simulink model "P2"  (R2018a)
settings: Solver=VariableStepAuto  StartTime=0.0  StopTime=300  RelTol=1e-3
values from neighbouring files (symbols this model uses):
  n = 5    [Q2.m]
undefined symbols (not defined in the file or in its folder): m
settings Model: Creator=aminrakhsha  LastModifiedBy=whitefox

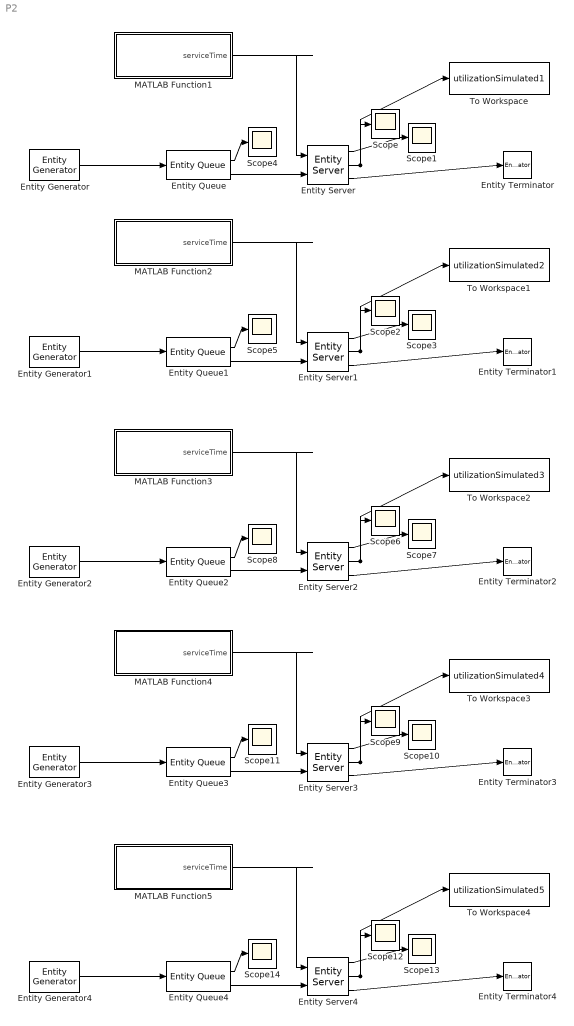
== system P2 ==
  Entity Generator : EntityGenerator  OutputPortMessageModes=m  TimeSource=MATLAB action  Period=5  IntergenerationTimeAction=|  EntityType=Structured  EntityTypeName=Entity
      | persistent counter;
      | if isempty(counter)
      |    counter = 1;
      | end 
      | if counter <= 100
      |     mean=2;
      |     dt = -mean*log(1-rand());
      | else
      |     dt = inf;
      | end
      | counter = counter + 1
  Entity Generator1 : EntityGenerator  OutputPortMessageModes=m  TimeSource=MATLAB action  Period=5  IntergenerationTimeAction=|  EntityType=Structured  EntityTypeName=Entity
      | persistent counter
      | if isempty(counter)
      |    counter = 1;
      | end 
      | if counter <= 100
      |     mean=2;
      |     dt = -mean*log(1-rand());
      | else
      |     dt = inf;
      | end
      | counter = counter + 1
  Entity Generator2 : EntityGenerator  OutputPortMessageModes=m  TimeSource=MATLAB action  Period=5  IntergenerationTimeAction=|  EntityType=Structured  EntityTypeName=Entity
      | persistent counter
      | if isempty(counter)
      |    counter = 1;
      | end 
      | if counter <= 100
      |     mean=2;
      |     dt = -mean*log(1-rand());
      | else
      |     dt = inf;
      | end
      | counter = counter + 1
  Entity Generator3 : EntityGenerator  OutputPortMessageModes=m  TimeSource=MATLAB action  Period=5  IntergenerationTimeAction=|  EntityType=Structured  EntityTypeName=Entity
      | persistent counter
      | if isempty(counter)
      |    counter = 1;
      | end 
      | if counter <= 100
      |     mean=2;
      |     dt = -mean*log(1-rand());
      | else
      |     dt = inf;
      | end
      | counter = counter + 1
  Entity Generator4 : EntityGenerator  OutputPortMessageModes=m  TimeSource=MATLAB action  Period=5  IntergenerationTimeAction=|  EntityType=Structured  EntityTypeName=Entity
      | persistent counter
      | if isempty(counter)
      |    counter = 1;
      | end 
      | if counter <= 100
      |     mean=2;
      |     dt = -mean*log(1-rand());
      | else
      |     dt = inf;
      | end
      | counter = counter + 1
  Entity Queue{,1..4} (5 alike) : EntityQueue  InputPortMessageModes=m  OutputPortMessageModes=n,m  Capacity=inf  AverageWait=on
      settings: OutputPortMap=o2,o5
  Entity Server{,1..4} (5 alike) : EntityServer  InputPortMessageModes=n,m  OutputPortMessageModes=n,n,m  Capacity=1  ServiceTimeSource=Signal port  ServiceTimeAttributeName=Attribute1  ServiceTimeAction=dt = getST(y);  AverageWait=on  Utilization=on
      settings: InputPortMap=u0,u2  OutputPortMap=o4,o5,o9
  Entity Terminator{,1..4} (5 alike) : EntityTerminator  InputPortMessageModes=m
  MATLAB Function1 : MATLAB Function  TreatAsAtomicUnit=on
  MATLAB Function2 : MATLAB Function  TreatAsAtomicUnit=on
  MATLAB Function3 : MATLAB Function  TreatAsAtomicUnit=on
  MATLAB Function4 : MATLAB Function  TreatAsAtomicUnit=on
  MATLAB Function5 : MATLAB Function  TreatAsAtomicUnit=on
  Scope{,1..14} (15 alike) : Scope
  To Workspace : ToWorkspace  VariableName=utilizationSimulated1  SaveFormat=Timeseries  SampleTime=-1
  To Workspace1 : ToWorkspace  VariableName=utilizationSimulated2  SaveFormat=Timeseries  SampleTime=-1
  To Workspace2 : ToWorkspace  VariableName=utilizationSimulated3  SaveFormat=Timeseries  SampleTime=-1
  To Workspace3 : ToWorkspace  VariableName=utilizationSimulated4  SaveFormat=Timeseries  SampleTime=-1
  To Workspace4 : ToWorkspace  VariableName=utilizationSimulated5  SaveFormat=Timeseries  SampleTime=-1
  wires:
  Entity Queue/2 -> Entity Server/2
  Entity Server/3 -> Entity Terminator/1
  Entity Server/1 -> Scope1/1
  Entity Queue/1 -> Scope4/1
  MATLAB Function1/1(serviceTime) -> Entity Server/1
  Entity Server/2 -> To Workspace/1, Scope/1
  Entity Server1/3 -> Entity Terminator1/1
  Entity Server1/2 -> To Workspace1/1, Scope2/1
  Entity Generator1/1 -> Entity Queue1/1
  Entity Server1/1 -> Scope3/1
  Entity Queue1/2 -> Entity Server1/2
  Entity Queue1/1 -> Scope5/1
  MATLAB Function2/1(serviceTime) -> Entity Server1/1
  Entity Server2/3 -> Entity Terminator2/1
  Entity Server2/2 -> To Workspace2/1, Scope6/1
  Entity Generator2/1 -> Entity Queue2/1
  Entity Server2/1 -> Scope7/1
  Entity Queue2/2 -> Entity Server2/2
  Entity Queue2/1 -> Scope8/1
  MATLAB Function3/1(serviceTime) -> Entity Server2/1
  Entity Server3/3 -> Entity Terminator3/1
  Entity Server3/2 -> To Workspace3/1, Scope9/1
  Entity Generator3/1 -> Entity Queue3/1
  Entity Server3/1 -> Scope10/1
  Entity Queue3/2 -> Entity Server3/2
  Entity Queue3/1 -> Scope11/1
  MATLAB Function4/1(serviceTime) -> Entity Server3/1
  Entity Server4/3 -> Entity Terminator4/1
  Entity Server4/2 -> To Workspace4/1, Scope12/1
  Entity Generator4/1 -> Entity Queue4/1
  Entity Server4/1 -> Scope13/1
  Entity Queue4/2 -> Entity Server4/2
  Entity Queue4/1 -> Scope14/1
  MATLAB Function5/1(serviceTime) -> Entity Server4/1
  Entity Generator/1 -> Entity Queue/1

== matlab function P2/MATLAB Function1 ==
  data: serviceTime output
function serviceTime = serviceTimeFunction()
    persistent counter
    if isempty(counter)
        counter = 1;
        rng(11)
    end 
    mu = 3;
    sigma = 0.2;
    serviceTime = normrnd(mu,sigma);

== matlab function P2/MATLAB Function2 ==
  data: serviceTime output
function serviceTime = serviceTimeFunction()
    persistent counter
    if isempty(counter)
        counter = 1;
        rng(19)
    end 
    mu = 3;
    sigma = 0.2;
    serviceTime = normrnd(mu,sigma);

== matlab function P2/MATLAB Function3 ==
  data: serviceTime output
function serviceTime = serviceTimeFunction()
    persistent counter
    if isempty(counter)
        counter = 1;
        rng(23)
    end 
    mu = 3;
    sigma = 0.2;
    serviceTime = normrnd(mu,sigma);

== matlab function P2/MATLAB Function4 ==
  data: serviceTime output
function serviceTime = serviceTimeFunction()
    persistent counter
    if isempty(counter)
        counter = 1;
        rng(29)
    end 
    mu = 3;
    sigma = 0.2;
    serviceTime = normrnd(mu,sigma);

== matlab function P2/MATLAB Function5 ==
  data: serviceTime output
function serviceTime = serviceTimeFunction()
    persistent counter
    if isempty(counter)
        counter = 1;
        rng(31)
    end 
    mu = 3;
    sigma = 0.2;
    serviceTime = normrnd(mu,sigma);
